simulink model "Senorless"  (R2023a)
settings: Solver=FixedStepDiscrete  StartTime=0.0  StopTime=2  FixedStep=1/FOC_FRQ  RelTol=1e-3
values from neighbouring files (symbols this model uses):
  ADC_REF = 3.6    [Senorless.sldd]
  ADC_SAMPLE_MAX = 32767.0    [Senorless.sldd]
  AMP_GAIN = 32.0    [Senorless.sldd]
  CURR_INPUT = 3276.0    [Senorless.sldd]
  CURR_KI = 380.0    [Senorless.sldd]
  CURR_KP = 0.04    [Senorless.sldd]
  CURR_LIMIT = 1.1    [Senorless.sldd]
  CURR_OVER = 34.0    [Senorless.sldd]
  CURR_POINT_GAIN = 7.0    [Senorless.sldd]
  CURR_STEP = 32760.0    [Senorless.sldd]
  CURR_UNDER = 0.03    [Senorless.sldd]
  CURR_WIDTH = 250.0    [Senorless.sldd]
  FOC_FRQ = 36000.0    [Senorless.sldd]
  GAMMA = 32767.0    [Senorless.sldd]
  HFI_ID = 2.125    [Senorless.sldd]
  IMAX = 34.0    [Senorless.sldd]
  LPF_FRQ = 300.0    [Senorless.sldd]
  MOTOR_DAMPER = 8.3E-7    [Senorless.sldd]
  MOTOR_FLUX = 0.0012713112    [Senorless.sldd]
  MOTOR_INERTIA = 1.02E-6    [Senorless.sldd]
  MOTOR_LS = 1.8E-5    [Senorless.sldd]
  MOTOR_PN = 7.0    [Senorless.sldd]
  MOTOR_RS = 0.065    [Senorless.sldd]
  NS_COMP_UD = 0.531    [Senorless.sldd]
  PLL_LIMIT = 0.95    [Senorless.sldd]
  PLL_WIDTH = 500.0    [Senorless.sldd]
  PWM_FRQ = 96000000.0    [Senorless.sldd]
  RS_HUNT = 0.002    [Senorless.sldd]
  SMOK_FRQ = 1200.0    [Senorless.sldd]
  SPD_LIMIT = 0.8    [Senorless.sldd]
  SPD_LPF_LEVEL = 15.0    [Senorless.sldd]
  SPD_MAX = 8100.0    [Senorless.sldd]
  SPD_MIN = -8100.0    [Senorless.sldd]
  SPD_REDUCE = 380.0    [Senorless.sldd]
  SPD_STEP = 3.0    [Senorless.sldd]
  SPD_WIDTH = 10.0    [Senorless.sldd]
  TS_POINT_GAIN = 10.0    [Senorless.sldd]
  UDC = 17.0    [Senorless.sldd]
  UDC_GAIN = 21.0    [Senorless.sldd]
  UDC_POINT_GAIN = 10.0    [Senorless.sldd]
undefined symbols (not defined in the file or in its folder): curr_q_ki, curr_q_kp, DiscIntNeverNeededParam, magnitude, PLL_LPF_LEVEL, Udc
libraries: simulink x20, slpidlib x5, mcbcontrolslib x4, mcbplantlib x1, autolibpmsminterior x1, autolibpmsmexterior x1, spspowerguiLib x1
(part 1 of 7)
settings Model: DataDictionary=Senorless.sldd  NumberOfSteps=10000  SnapshotBufferSize=5000  SnapshotInterval=5000  PacingRate=0.100000  Creator=lzm  LastModifiedBy=liangzhuoming
settings DataIOCC: SaveFormat=StructureWithTime  DSMLogging=off  ReturnWorkspaceOutputs=off
settings OptimizationCC: DefaultParameterBehavior=Inlined  GainParamInheritBuiltInType=on  UseFloatMulNetSlope=on  InheritOutputTypeSmallerThanSingle=on  DefaultUnderspecifiedDataType=single  UseSpecifiedMinMax=on  InlineInvariantSignals=on  StrengthReduction=on  PassReuseOutputArgsAs=Individual arguments  ZeroExternalMemoryAtStartup=off  ZeroInternalMemoryAtStartup=off  NoFixptDivByZeroProtection=on  EfficientFloat2IntCast=on  LifeSpan=1  OptimizeBlockOrder=speed  OptimizationPriority=Speed  MultiThreadedLoops=on  EfficientTunableParamExpr=on
settings DebuggingCC: SignalRangeChecking=warning  ParameterTunabilityLossMsg=error  UnconnectedInputMsg=warning  UnconnectedOutputMsg=warning  UnconnectedLineMsg=warning
settings HardwareCC: ProdBitPerPointer=32  ProdBitPerSizeT=32  ProdBitPerPtrDiffT=32  ProdLargestAtomicInteger=Long  ProdLargestAtomicFloat=Double  ProdWordSize=32  ProdLongLongMode=on  ProdHWDeviceType=ARM Compatible->ARM Cortex-M
settings ModelReferenceCC: EnableRefExpFcnMdlSchedulingChecks=on
settings SFSimCC: MATLABDynamicMemAlloc=off
settings RTWCC: Description=Embedded Coder  SystemTargetFile=ert.tlc  GenCodeOnly=on  TemplateMakefile=ert_default_tmf  GenerateReport=on  BuildConfiguration=Faster Runs  LaunchReport=on  GenerateCodeReplacementReport=on  DLArmComputeVersion=19.05
settings CodeAppCC: ForceParamTrailComments=on  IgnoreCustomStorageClasses=off  OperatorAnnotations=on  SimulinkDataObjDesc=on  SFDataObjDesc=on  CustomSymbolStrGlobalVar=rt$N$M  CustomSymbolStrType=$N$M  CustomSymbolStrFcn=$N$M$F  CustomSymbolStrMacro=$N$M  InsertBlockDesc=on
settings ERTTargetCC: TargetLangStandard=C99 (ISO)  GenerateSampleERTMain=on  IncludeMdlTerminateFcn=off  CombineSignalStateStructs=on  SupportNonFinite=off  SupportComplex=off  SupportNonInlinedSFcns=on  InlinedParameterPlacement=NonHierarchical  ERTCustomFileTemplate=example_file_process.tlc  ERTFilePackagingFormat=CompactWithDataFile

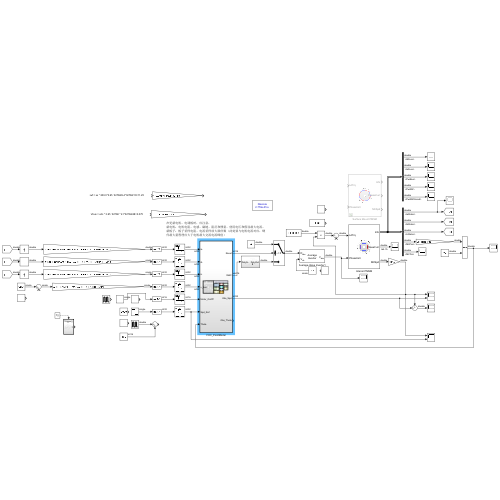
[thumbnail: Simulink's stored preview of the top-level diagram]
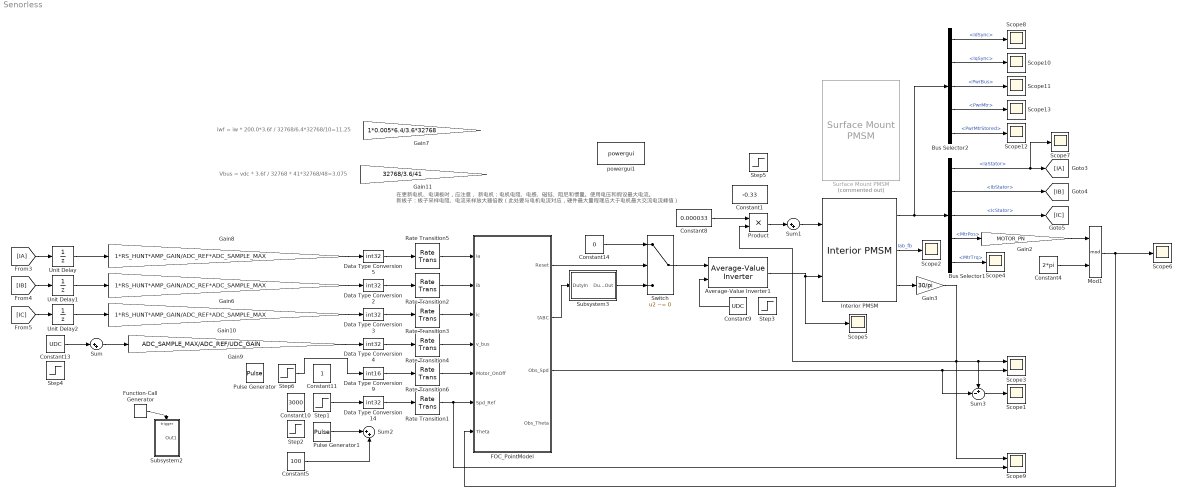
== system Senorless ==
  note: 在更新电机、电调板时，应注意，
      | 新电机：电机电阻、电感、磁链、阻尼和惯量。使用电压和假设最大电流。
      | 新板子：板子采样电阻、电流采样放大器倍数（此处要与电机电流对应，硬件最大量程理应大于电机最大交流电流峰值）
  note: iwf = iw * 200.0*3.6f / 32768/6.4*32768/10=11.25
  note: Vbus = vdc * 3.6f / 32768 * 41*32768/48=3.075
  Average-Value Inverter1 : mcbplantlib/Average-Value Inverter
  Bus Selector1 : BusSelector  OutputSignals=IaStator,IbStator,IcStator,MtrPos,MtrTrq
  Bus Selector2 : BusSelector  OutputSignals=IdSync,IqSync,PwrInfo.PwrTrnsfrd.PwrBus,PwrInfo.PwrTrnsfrd.PwrMtr,PwrInfo.PwrStored.PwrMtrStored
  Constant1 : Constant  Value=-0.33
  Constant10 : Constant  Value=3000  OutDataTypeStr=int16
  Constant11 : Constant
  Constant13 : Constant  Value=UDC  OutDataTypeStr=single
  Constant14 : Constant  Value=0
  Constant4 : Constant  Value=2*pi
  Constant5 : Constant  Value=100  OutDataTypeStr=int16
  Constant8 : Constant  Value=0.000033
  Constant9 : Constant  Value=UDC
  Data Type Conversion{2..5,14} (5 alike) : DataTypeConversion  OutDataTypeStr=int32  SaturateOnIntegerOverflow=off  RndMeth=Floor
  Data Type Conversion9 : DataTypeConversion  OutDataTypeStr=int16  SaturateOnIntegerOverflow=off  RndMeth=Floor
  FOC_PointModel : Subsystem  TreatAsAtomicUnit=on
      settings: RTWSystemCode=Nonreusable function
  Function-Call Generator : simulink/Ports & Subsystems/Function-Call Generator  sample_time=1/2500*100  numberOfIterations=1  DisallowWideOutput=off
  Gain10 : Gain  Gain=1*RS_HUNT*AMP_GAIN/ADC_REF*ADC_SAMPLE_MAX  OutDataTypeStr=single
  Gain11 : Gain  Gain=32768/3.6/41
  Gain2 : Gain  Gain=MOTOR_PN
  Gain3 : Gain  Gain=30/pi
  Gain6 : Gain  Gain=1*RS_HUNT*AMP_GAIN/ADC_REF*ADC_SAMPLE_MAX  OutDataTypeStr=single
  Gain7 : Gain  Gain=1*0.005*6.4/3.6*32768
  Gain8 : Gain  Gain=1*RS_HUNT*AMP_GAIN/ADC_REF*ADC_SAMPLE_MAX
  Gain9 : Gain  Gain=ADC_SAMPLE_MAX/ADC_REF/UDC_GAIN
  Interior PMSM : autolibpmsminterior/Interior PMSM  port_config=Torque  sim_type=Discrete  Ts=1/FOC_FRQ  FilePath=interiorpmsm_motordata.m  P=MOTOR_PN  Rs=MOTOR_RS  Ldq=[MOTOR_LS*0.7 MOTOR_LS/0.7]  KConstText=Permanent flux linkage constant (lambda_pm):  lambda_pm=MOTOR_FLUX  Ke=159.9771  mechanical=[MOTOR_INERTIA, MOTOR_DAMPER, 1e-6]  idq0=[0 0]  theta_init=1/MOTOR_PN*2*pi/360*0  omega_init=0  KConst=MOTOR_FLUX  lambda_pm_calc=MOTOR_FLUX  Kt=1.323  RefBlkName='autolibpmsminterior/Interior PMSM'  aMode=1
      settings: LibrarySourceBlock=autolibemachines/Interior PMSM
  Mod1 : Math  Operator=mod
  Product : Product
  Pulse Generator : DiscretePulseGenerator  PulseType=Time based  Period=1  PulseWidth=98
  Pulse Generator1 : DiscretePulseGenerator  PulseType=Time based  Amplitude=8100  Period=0.5  PulseWidth=90
  Rate Transition{1..6} (6 alike) : RateTransition
  Scope{1..2,4..8,10..13} (11 alike) : Scope
  Scope3 : Scope  NumInputPorts=2
  Scope9 : Scope  NumInputPorts=2
  Step1 : Step  Before=1000  After=-1000  OutDataTypeStr=single  SampleTime=0
  Step2 : Step  Time=1.5  After=8000  OutDataTypeStr=single  SampleTime=0
  Step3 : Step  Time=2.5  Before=48  After=47  OutDataTypeStr=single  SampleTime=0
  Step4 : Step  Time=2.5  Before=48  After=47  OutDataTypeStr=single  SampleTime=0
  Step5 : Step  Before=0.2  After=0  SampleTime=0
  Step6 : Step  Time=0.2  OutDataTypeStr=single  SampleTime=0
  Subsystem2 : Subsystem
  Subsystem3 : Subsystem
  Sum : Sum  Inputs=|++
  Sum1 : Sum  Inputs=|++
  Sum2 : Sum  Inputs=|++
  Sum3 : Sum  Inputs=+-|
  Surface Mount PMSM : autolibpmsmexterior/Surface Mount PMSM  Commented=on  port_config=Torque  sim_type=Discrete  Ts=1/FOC_FRQ  P=MOTOR_PN  Rs=MOTOR_RS  Ldq_=MOTOR_LS  KConstText=Permanent flux linkage constant (lambda_pm):  lambda_pm=MOTOR_FLUX  Ke=0.0059268  Kt=0.061  mechanical=[MOTOR_INERTIA, MOTOR_DAMPER, 0]  idq0=[0 0]  theta_init=4/5  omega_init=0  KConst=MOTOR_FLUX  lambda_pm_calc=MOTOR_FLUX  RefBlkName='autolibpmsmexterior/Surface Mount PMSM'  aMode=5  Ldq="[0.0017      0.0017]"
  Switch : Switch  Criteria=u2 ~= 0  SaturateOnIntegerOverflow=off  InputSameDT=off
  Unit Delay : UnitDelay  SampleTime=-1  HasFrameUpgradeWarning=on
  Unit Delay1 : UnitDelay  SampleTime=-1  HasFrameUpgradeWarning=on
  Unit Delay2 : UnitDelay  SampleTime=-1  HasFrameUpgradeWarning=on
  powergui1 : spspowerguiLib/powergui  Priority=1  SimulationMode=Discrete  SampleTime=1/FOC_FRQ  frequency=60  Iterations=50  frequencyindice=60  Pbase=100e6  ErrMax=1e-4  UnitsV=kV  UnitsW=MW  buscounter=0  FunctionMessages=off  echomessages=off  EnableUseOfTLC=off  CurrentSourceSwitches=off  DisableSnubberDevices=off  DisableRonSwitches=off  DisableVfSwitches=off  DisplayEquations=off  AutomaticDiscreteSolvers=off  SolverType=Tustin/Backward Euler (TBE)  Interpol=off  ExternalGateDelay=off  methode=off  Ts=100  x0status=blocks  SPID=on  SwTol=0  HookPort=off  NonlinearTolerance=1e-4  nMaxIteration=100  ContinueOnMaxIteration=off  RestoreLinks=warning  ResistiveCurrentMeasurement=off  Frange=[0:2:500]  Ylog=off  Xlog=on  ShowGrid=off  save=off  variable=ZData  structure=0  ZoomFFT=off  StartTime=0.0  cycles=1  DisplayStyle=1  fundamental=60  FreqAxis=off  MaxFrequency=1000  frequencyindicesteady=1  RmsSteady=1  display=off
  wires:
  Interior PMSM/3 -> Gain3/1
  Interior PMSM/2 -> Scope2/1  "Iab_fb"
  Interior PMSM/1 -> Bus Selector2/1, Bus Selector1/1
  Bus Selector1/1 -> Scope7/1, [IA]  "<IaStator>"
  Constant4/1 -> Mod1/2
  Gain2/1 -> Mod1/1
  Bus Selector1/4 -> Gain2/1  "<MtrPos>"
  Data Type Conversion5/1 -> Rate Transition5/1
  Data Type Conversion2/1 -> Rate Transition2/1
  Data Type Conversion3/1 -> Rate Transition3/1
  Data Type Conversion9/1 -> Rate Transition6/1
  [IC] -> Unit Delay2/1
  Gain8/1 -> Data Type Conversion5/1
  Gain6/1 -> Data Type Conversion2/1
  Gain10/1 -> Data Type Conversion3/1
  Gain9/1 -> Data Type Conversion4/1
  [IB] -> Unit Delay1/1
  [IA] -> Unit Delay/1
  FOC_PointModel/2(tABC) -> Subsystem3/1(DutyIn)
  Gain3/1 -> Scope9/1, Scope3/1, Sum3/1, Product/2
  Sum/1 -> Gain9/1
  Data Type Conversion4/1 -> Rate Transition4/1
  Mod1/1 -> FOC_PointModel/7(Theta), Scope6/1
  FOC_PointModel/3(Obs_Spd) -> Sum3/2, Scope3/2
  Data Type Conversion14/1 -> Rate Transition1/1
  Subsystem3/1(DutyOut) -> Switch/3
  Bus Selector1/5 -> Scope4/1  "<MtrTrq>"
  Average-Value Inverter1/1 -> Scope5/1, Interior PMSM/2
  FOC_PointModel/1(Reset) -> Switch/2
  Constant14/1 -> Switch/1
  Constant9/1 -> Average-Value Inverter1/2
  Constant13/1 -> Sum/1
  Rate Transition1/1 -> Scope9/2, FOC_PointModel/6(Spd_Ref)
  Function-Call Generator/1 -> Subsystem2/Trigger
  Rate Transition5/1 -> FOC_PointModel/1(ia)
  Rate Transition2/1 -> FOC_PointModel/2(ib)
  Rate Transition3/1 -> FOC_PointModel/3(ic)
  Rate Transition4/1 -> FOC_PointModel/4(v_bus)
  Rate Transition6/1 -> FOC_PointModel/5(Motor_OnOff)
  Constant5/1 -> Sum2/2
  Pulse Generator1/1 -> Sum2/1
  Constant8/1 -> Product/1
  Product/1 -> Sum1/1
  Bus Selector1/3 -> [IC]  "<IcStator>"
  Bus Selector1/2 -> [IB]  "<IbStator>"
  Switch/1 -> Average-Value Inverter1/1
  Sum3/1 -> Scope1/1
  Unit Delay/1 -> Gain8/1
  Unit Delay1/1 -> Gain6/1
  Unit Delay2/1 -> Gain10/1
  Bus Selector2/1 -> Scope8/1  "<IdSync>"
  Bus Selector2/2 -> Scope10/1  "<IqSync>"
  Bus Selector2/3 -> Scope11/1  "<PwrBus>"
  Bus Selector2/4 -> Scope13/1  "<PwrMtr>"
  Bus Selector2/5 -> Scope12/1  "<PwrMtrStored>"
  Step6/1 -> Data Type Conversion9/1
  Step1/1 -> Data Type Conversion14/1
  Sum1/1 -> Interior PMSM/1

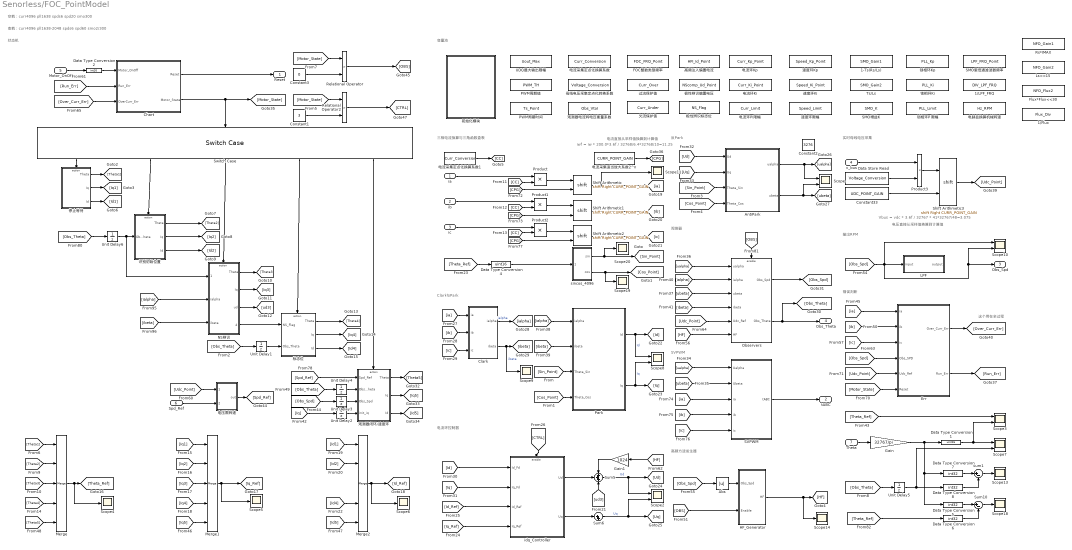
== system Senorless/FOC_PointModel ==
  note: 高频方波发生器
  note: 输出RPM
  note: 空载：curr4096 pll1638 spds6 spd20 smo300
  note: 这个用在全过程
  note: 错误判断
  note: 观测器
  note: SVPWM
  note: 反Park
  note: 实时母线电压采集
  note: 电流环控制器
  note: Clark与Park
  note: 三相电流换算与三角函数查表
  note: 变量池
  note: 状态机
  note: 电流直接从采样值换算到计算值
  note: Vbus = vdc * 3.6f / 32767 * 41*32767/48=3.075
  note: iwf = iw * 200.0*3.6f / 32768/6.4*32768/10=11.25
  note: 电压直接从采样值换算到计算值
  note: 变载：curr4096 pll1638-2048 spds6 spd60 smo2/300
  ia : Inport  OutDataTypeStr=int32
  ib : Inport  Port=2  OutDataTypeStr=int32
  ic : Inport  Port=3  OutDataTypeStr=int32
  v_bus : Inport  Port=4  OutDataTypeStr=int32
  Motor_OnOff : Inport  Port=5
  Spd_Ref : Inport  Port=6
  Theta : Inport  Port=7
  1-Ts(Rs/Ls) : DataStoreMemory  DataStoreName=SMO_Gain1  WriteAfterWriteMsg=warning  ShowAdditionalParam=off
  1/Flux : DataStoreMemory  DataStoreName=Flux_Div  WriteAfterWriteMsg=warning  ShowAdditionalParam=off
  1/LPF_FRQ : DataStoreMemory  DataStoreName=DIV_LPF_FRQ  WriteAfterWriteMsg=warning  ShowAdditionalParam=off
  Abs : Abs  SaturateOnIntegerOverflow=off
  AntiPark : Subsystem
  Chart : Stateflow chart  TreatAsAtomicUnit=on
  Clark : Subsystem
  Constant1 : Constant  Value=3  OutDataTypeStr=uint8
  Constant2 : Constant  Value=3276  OutDataTypeStr=int16
  Constant3 : Constant  Value=0  OutDataTypeStr=uint8
  Constant33 : Constant  Value=UDC_POINT_GAIN
  Data Store Read : DataStoreRead  DataStoreName=Voltage_Conversion  IndexOptions=Index vector (dialog)  Indices=1  OutputSizes=1
  Data Type Conversion1 : DataTypeConversion  OutDataTypeStr=uint16  SaturateOnIntegerOverflow=off  RndMeth=Floor
  Data Type Conversion2 : DataTypeConversion  OutDataTypeStr=int16  SaturateOnIntegerOverflow=off
  Data Type Conversion4 : DataTypeConversion  OutDataTypeStr=uint16  SaturateOnIntegerOverflow=off
  Data Type Conversion{5..8} (4 alike) : DataTypeConversion  OutDataTypeStr=int32  SaturateOnIntegerOverflow=off
  Err : Subsystem
  FOC整数类型频率 : DataStoreMemory  DataStoreName=FOC_FRQ_Point  WriteAfterWriteMsg=warning  ShowAdditionalParam=off
  Flux*Flux<<30 : DataStoreMemory  DataStoreName=NFO_Flux2  WriteAfterWriteMsg=warning  ShowAdditionalParam=off
  Gain : Gain  Gain=32767/pi
  Gain1 : Gain  Gain=1024  ParamDataTypeStr=int16  OutDataTypeStr=int16  RndMeth=Zero
  HF_Generator : Subsystem
  LPF : Subsystem  TreatAsAtomicUnit=on
  Ls<<15 : DataStoreMemory  DataStoreName=NFO_Gain2  WriteAfterWriteMsg=warning  ShowAdditionalParam=off
  Merge : Merge  Inputs=5
  Merge1 : Merge  Inputs=5
  Merge2 : Merge  Inputs=5
  NS辨识 : Subsystem  TreatAsAtomicUnit=on
  Observers : Subsystem
  PWM周期值 : DataStoreMemory  DataStoreName=PWM_TH  WriteAfterWriteMsg=warning  ShowAdditionalParam=off
  PWM周期时间 : DataStoreMemory  DataStoreName=Ts_Point  WriteAfterWriteMsg=warning  ShowAdditionalParam=off
  Park : Subsystem
  Product{,1..3} (4 alike) : Product  OutDataTypeStr=int32  RndMeth=Zero
  Relational Operator : RelationalOperator  Operator=>  OutDataTypeStr=boolean  RndMeth=Zero  InputSameDT=off
  Relational Operator2 : RelationalOperator  Operator=>  OutDataTypeStr=boolean  RndMeth=Zero  InputSameDT=off
  Rs*IMAX : DataStoreMemory  DataStoreName=NFO_Gain1  WriteAfterWriteMsg=warning  ShowAdditionalParam=off
  SMO增益K : DataStoreMemory  DataStoreName=SMO_K  WriteAfterWriteMsg=warning  ShowAdditionalParam=off
  SMO里低通滤波器频率 : DataStoreMemory  DataStoreName=LPF_FRQ_Point  WriteAfterWriteMsg=warning  ShowAdditionalParam=off
  SVPWM : Subsystem  ScheduleAs=Aperiodic partition  PartitionName=TEMP_PRECOMP_PARTITION_NAME_MessageTriggeredSubsystem
  Scope{,2..3,7..8,10} (6 alike) : Scope  NumInputPorts=2
  Scope{4..6,9,11,13..14,18..20} (10 alike) : Scope
  Shift Arithmetic{,1..3} (4 alike) : ArithShift  BitShiftNumberSource=Input port  BitShiftNumber=CURR_POINT_GAIN  BitShiftDirection=Right
      settings: InputPortMap=u0,p1
  Sum1 : Sum  Inputs=|+-  OutDataTypeStr=int32
  Sum10 : Sum  Inputs=|+-  OutDataTypeStr=int32
  Sum5 : Sum  Inputs=+++
  Sum6 : Sum  Inputs=|++
  Switch Case : SwitchCase  CaseConditions={0,1,2,3,4}  ShowDefaultCase=off
  Ts/Ls : DataStoreMemory  DataStoreName=SMO_Gain2  WriteAfterWriteMsg=warning  ShowAdditionalParam=off
  UDQ最大输出限幅 : DataStoreMemory  DataStoreName=Uout_Max  WriteAfterWriteMsg=warning  ShowAdditionalParam=off
  Unit Delay{1..6} (6 alike) : UnitDelay  SampleTime=-1  HasFrameUpgradeWarning=on
  idq_Controller : Subsystem
  sincos_4096 : Subsystem
  停止等待 : Subsystem  TreatAsAtomicUnit=on
  初始化模块 : Subsystem  TreatAsAtomicUnit=on
  极性辨识偏置电压 : DataStoreMemory  DataStoreName=NScomp_Ud_Point  WriteAfterWriteMsg=warning  ShowAdditionalParam=off
  极性辨识标志位 : DataStoreMemory  DataStoreName=NS_Flag  WriteAfterWriteMsg=warning  ShowAdditionalParam=off
  标志位 : Subsystem  TreatAsAtomicUnit=on
  欠流保护值 : DataStoreMemory  DataStoreName=Curr_Under  WriteAfterWriteMsg=warning  ShowAdditionalParam=off
  母线电压采集定点化转换系数 : DataStoreMemory  DataStoreName=Voltage_Conversion  WriteAfterWriteMsg=warning  ShowAdditionalParam=off
  电压限转速 : Subsystem
  电流环Ki : DataStoreMemory  DataStoreName=Curr_Ki_Point  WriteAfterWriteMsg=warning  ShowAdditionalParam=off
  电流环Kp : DataStoreMemory  DataStoreName=Curr_Kp_Point  WriteAfterWriteMsg=warning  ShowAdditionalParam=off
  电流环PI限幅 : DataStoreMemory  DataStoreName=Curr_Limit  WriteAfterWriteMsg=warning  ShowAdditionalParam=off
  电流采集定点化换算系数 : DataStoreMemory  DataStoreName=Curr_Conversion  WriteAfterWriteMsg=warning  ShowAdditionalParam=off
  电流采集定点化换算系数1 : DataStoreRead  DataStoreName=Curr_Conversion  IndexOptions=Index vector (dialog)  Indices=1  OutputSizes=1
  电流采集适当放大系数2^n : Constant  Value=CURR_POINT_GAIN
  电赫兹换算机械转速 : DataStoreMemory  DataStoreName=Hz_RPM  WriteAfterWriteMsg=warning  ShowAdditionalParam=off
  观测器电流转电压衡量系数 : DataStoreMemory  DataStoreName=Obs_VtoI  WriteAfterWriteMsg=warning  ShowAdditionalParam=off
  观测器闭环/速度环 : Subsystem  TreatAsAtomicUnit=on
  识别初始位置 : Subsystem  TreatAsAtomicUnit=on
  过流保护值 : DataStoreMemory  DataStoreName=Curr_Over  WriteAfterWriteMsg=warning  ShowAdditionalParam=off
  速度环Ki : DataStoreMemory  DataStoreName=Speed_Ki_Point  WriteAfterWriteMsg=warning  ShowAdditionalParam=off
  速度环Kp : DataStoreMemory  DataStoreName=Speed_Kp_Point  WriteAfterWriteMsg=warning  ShowAdditionalParam=off
  速度环限幅 : DataStoreMemory  DataStoreName=Speed_Limit  WriteAfterWriteMsg=warning  ShowAdditionalParam=off
  锁相环Ki : DataStoreMemory  DataStoreName=PLL_Ki  WriteAfterWriteMsg=warning  ShowAdditionalParam=off
  锁相环Kp : DataStoreMemory  DataStoreName=PLL_Kp  WriteAfterWriteMsg=warning  ShowAdditionalParam=off
  锁相环PI限幅 : DataStoreMemory  DataStoreName=PLL_Limit  WriteAfterWriteMsg=warning  ShowAdditionalParam=off
  高频注入偏置电流 : DataStoreMemory  DataStoreName=HFI_Id_Point  WriteAfterWriteMsg=warning  ShowAdditionalParam=off
  Reset : Outport
  tABC : Outport  Port=2
  Obs_Spd : Outport  Port=3
  Obs_Theta : Outport  Port=4
  wires:
  Motor_OnOff/1 -> Data Type Conversion2/1
  Switch Case/1 -> 停止等待/Action
  Switch Case/3 -> NS辨识/Action
  Switch Case/2 -> 识别初始位置/Action
  Switch Case/4 -> 标志位/Action
  [Sin_Point] -> AntiPark/3(Theta_Sin)
  [Cos_Point] -> AntiPark/4(Theta_Cos)
  v_bus/1 -> Product3/1
  Product1/1 -> Shift Arithmetic1/1
  Product2/1 -> Shift Arithmetic2/1
  电流采集定点化换算系数1/1 -> [CC]
  [CC] -> Product/2
  [CC] -> Product1/2
  Data Store Read/1 -> Product3/2
  Unit Delay1/1 -> 标志位/2(Obs_Theta)
  停止等待/1(Theta) -> [Theta1]
  停止等待/2(Iq) -> [Iq1]
  停止等待/3(Id) -> [Id1]
  识别初始位置/1(Theta) -> [Theta2]
  识别初始位置/2(Iq) -> [Iq2]
  识别初始位置/3(Id) -> [Id2]
  标志位/2(Iq) -> [Iq4]
  标志位/3(Id) -> [Id4]
  [Theta1] -> Merge/1
  [Theta3] -> Merge/3
  [Theta4] -> Merge/4
  [Iq1] -> Merge1/1
  [Iq2] -> Merge1/2
  [Iq3] -> Merge1/3
  [Iq4] -> Merge1/4
  Merge1/1 -> [Iq_Ref], Scope5/1
  [Id1] -> Merge2/1
  [Id2] -> Merge2/2
  [Id4] -> Merge2/4
  [Iq_Ref] -> idq_Controller/4(Iq_Ref)
  Shift Arithmetic/1 -> [ia], Scope11/1
  Shift Arithmetic1/1 -> [ib]
  Shift Arithmetic2/1 -> [ic]
  [ia] -> Clark/1(ia)
  [ib] -> Clark/2(ib)
  [ic] -> Clark/3(ic)
  [Iq] -> idq_Controller/2(Iq_Fd)
  [Id] -> idq_Controller/1(Id_Fd)
  [ualpha] -> SVPWM/1(Ualpha)
  [ubeta] -> SVPWM/2(Ubeta)
  Clark/1(ialpha) -> [ialpha]  "ialpha"
  Clark/2(ibeta) -> Scope9/1, [ibeta]  "ibeta"
  [ualpha] -> Observers/1(ualpha)
  [ibeta] -> Observers/4(ibeta)
  [ubeta] -> Observers/3(ubeta)
  [ialpha] -> Observers/2(ialpha)
  标志位/1(Theta) -> [Theta4]
  Observers/2(Obs_Theta) -> Obs_Theta/1, [Obs_Theta]
  Switch Case/5 -> 观测器闭环/速度环/Action
  观测器闭环/速度环/2(Iq) -> [Iq5]
  观测器闭环/速度环/3(Id) -> [Id5]
  [Iq5] -> Merge1/5
  [Id5] -> Merge2/5
  Theta/1 -> Gain/1
  [Theta5] -> Merge/5
  Gain/1 -> Data Type Conversion5/1, Data Type Conversion7/1, Data Type Conversion1/1
  [Theta_Ref] -> Data Type Conversion4/1
  Chart/2(Motor_State) -> Switch Case/1, [Motor_State]
  Merge/1 -> Scope4/1, [Theta_Ref]
  Sum1/1 -> Scope13/1
  Data Type Conversion7/1 -> Sum1/1
  Data Type Conversion8/1 -> Sum1/2
  [Obs_Theta] -> Unit Delay5/1
  [CC] -> Product2/2
  Product3/1 -> Shift Arithmetic3/1
  Constant33/1 -> Shift Arithmetic3/2
  [Theta_Ref] -> Scope3/1
  [Obs_Spd] -> Unit Delay3/1
  [Run_Err] -> Chart/2(Run_Err)
  SVPWM/1(tABC) -> tABC/1
  Chart/1(Reset) -> Reset/1
  [Obs_Theta] -> Unit Delay4/1
  Unit Delay3/1 -> 观测器闭环/速度环/3(Obs_Spd)
  Shift Arithmetic3/1 -> [Udc_Point]
  [Udc_Point] -> 电压限转速/1(Udc_Ref)
  [Over_Curr_Err] -> Chart/3(OverCurr_Err)
  ia/1 -> Product/1
  ic/1 -> Product2/1
  Data Type Conversion2/1 -> Chart/1(Motor_OnOff)
  Sum5/1 -> [Ud], Scope2/1  "Ud"
  [ia] -> Err/1(ia)
  [ib] -> Err/2(ib)
  [ic] -> Err/3(ic)
  [Obs_Spd] -> Err/4(Obs_SPD)
  Err/1(Over_Curr_Err) -> [Over_Curr_Err]
  Err/2(Run_Err) -> [Run_Err]
  [Motor_State] -> Err/6(Reset)
  [Udc_Point] -> Observers/5(Udc_Ref)
  [Udc_Point] -> Err/5(Udc_Ref)
  AntiPark/1(ualpha) -> Scope/1, [ualpha]
  AntiPark/2(ubeta) -> Scope/2, [ubeta]
  [ia] -> SVPWM/3(ia)
  [ib] -> SVPWM/4(ib)
  [ic] -> SVPWM/5(ic)
  [CPG] -> Shift Arithmetic/2
  [CPG] -> Shift Arithmetic1/2
  [CPG] -> Shift Arithmetic2/2
  Product/1 -> Shift Arithmetic/1
  电流采集适当放大系数2^n/1 -> [CPG]
  Relational Operator/1 -> [OBS]
  [Motor_State] -> Relational Operator/1
  Constant3/1 -> Relational Operator/2
  Park/1(Id) -> Scope8/1, [Id]  "Id"
  Park/2(Iq) -> Scope8/2, [Iq]  "Iq"
  [ialpha] -> Park/1(ialpha)
  [ibeta] -> Park/2(ibeta)
  [Sin_Point] -> Park/3(Theta_Sin)
  [Cos_Point] -> Park/4(Theta_Cos)
  Unit Delay5/1 -> Data Type Conversion8/1, Scope7/2
  ib/1 -> Product1/1
  Data Type Conversion6/1 -> Sum10/2
  Data Type Conversion5/1 -> Sum10/1
  [Theta_Ref] -> Data Type Conversion6/1
  Sum10/1 -> Scope18/1
  Data Type Conversion4/1 -> sincos_4096/1(theta)
  sincos_4096/2(cos) -> Scope19/1, [Cos_Point]
  sincos_4096/1(sin) -> Scope20/1, [Sin_Point]
  [Obs_Spd] -> LPF/1(input), Scope10/2, Obs_Spd/1, Scope10/1
  [Ud] -> AntiPark/1(Ud)
  [HF] -> Gain1/1
  idq_Controller/2(Uq) -> Sum6/1
  Spd_Ref/1 -> 电压限转速/2(SPD_Ref)
  [HF] -> Observers/6(HF)
  Observers/1(Obs_Spd) -> [Obs_Spd]
  电压限转速/1(out) -> [Spd_Ref]
  [Obs_Spd] -> Abs/1
  NS辨识/1(Theta) -> [Theta3]
  NS辨识/2(Iq) -> [Iq3]
  观测器闭环/速度环/1(Theta) -> [Theta5]
  Unit Delay4/1 -> 观测器闭环/速度环/2(Obs_Theta)
  [Theta2] -> Merge/2
  [Uq] -> AntiPark/2(Uq)
  Sum6/1 -> [Uq], Scope2/2  "Uq"
  HF_Generator/1(HF) -> Scope14/1, [HF]
  idq_Controller/1(Ud) -> Sum5/2
  Unit Delay6/1 -> NS辨识/1(Obs_Theta), 识别初始位置/1(Obs_Theta)
  Data Type Conversion1/1 -> Scope3/2, Scope7/1
  [Id_Ref] -> idq_Controller/3(Id_Ref)
  NS辨识/3(ud) -> [ud3]
  Gain1/1 -> Sum5/1
  Merge2/1 -> [Id_Ref], Scope6/1
  [Obs_Theta] -> Unit Delay6/1
  [ialpha] -> NS辨识/2(ialpha)
  [ibeta] -> NS辨识/3(ibeta)
  NS辨识/4(NS_Flag) -> 标志位/1(NS_Flag)
  [Obs_Theta] -> Unit Delay1/1
  [OBS] -> Observers/Enable
  Constant1/1 -> Relational Operator2/2
  [Motor_State] -> Relational Operator2/1
  Relational Operator2/1 -> [CTRL]
  [CTRL] -> idq_Controller/Enable
  [ud3] -> Sum5/3
  Abs/1 -> HF_Generator/1(Obs_Spd)
  [Iq] -> Unit Delay2/1
  Unit Delay2/1 -> 观测器闭环/速度环/4(init_iq)
  [Spd_Ref] -> 观测器闭环/速度环/1(Spd_Ref)
  [OBS] -> HF_Generator/2(Enable)

== system Senorless/Subsystem2 ==
  Trigger : TriggerPort  TriggerType=function-call  VariantControl=(inherit)  PortDimensions=1
  Constant1 : Constant  Value=0.25  OutDataTypeStr=single
  Constant16 : Constant  Value=SPD_MAX
  Product2 : Product
  Random Number1 : RandomNumber  Mean=0.1  Variance=0.01  Seed=15
  Saturation1 : Saturate  UpperLimit=1  LowerLimit=0
  Scope : Scope  NumInputPorts=2
  Sum : Sum  Inputs=|++
  Out1 : Outport
  wires:
  Saturation1/1 -> Product2/1
  Constant16/1 -> Product2/2
  Product2/1 -> Out1/1
  Sum/1 -> Scope/2, Saturation1/1
  Random Number1/1 -> Scope/1, Sum/1
  Constant1/1 -> Sum/2

== system Senorless/Subsystem3 ==
  DutyIn : Inport
  Constant : Constant  Value=0.5  SampleTime=-1
  Constant1 : Constant  SampleTime=-1
  Constant7 : Constant  Value=PWM_FRQ
  Constant8 : Constant  Value=FOC_FRQ*2
  Display : Display
  Divide : Product  Inputs=*/
  Divide1 : Product  Inputs=*/
  Divide2 : Product  Inputs=*/
  DutyIn1 : InportShadow
  Gain1 : Gain  Gain=-1
  Product : Product
  Scope : Scope  NumInputPorts=2
  Sum : Sum  Inputs=|+-
  Sum1 : Sum  Inputs=|++
  DutyOut : Outport
  wires:
  Divide/1 -> Product/1, Display/1
  Constant1/1 -> Divide/1
  Divide2/1 -> Divide1/2, Divide/2
  Constant7/1 -> Divide2/1
  Constant8/1 -> Divide2/2
  Product/1 -> Sum/1
  Sum1/1 -> DutyOut/1, Scope/2
  Gain1/1 -> Sum1/1
  DutyIn/1 -> Product/2
  Constant/1 -> Sum/2, Sum1/2
  Sum/1 -> Gain1/1
  Divide1/1 -> Scope/1
  DutyIn1/1 -> Divide1/1

== system Senorless/FOC_PointModel/AntiPark ==
  note: Valpha = ud*cos(theta) - uq*sin(theta);
      | Vbeta = ud*sin(theta) + uq*cos(theta);
  Ud : Inport
  Uq : Inport  Port=2
  Theta_Sin : Inport  Port=3
  Theta_Cos : Inport  Port=4
  Add : Sum  Inputs=+-  OutDataTypeStr=int32
  Add1 : Sum  OutDataTypeStr=int32
  Product{,1..3} (4 alike) : Product  OutDataTypeStr=int32  RndMeth=Zero
  Shift Arithmetic : ArithShift  BitShiftNumber=15  DiagnosticForOORShift=Error
  Shift Arithmetic1 : ArithShift  BitShiftNumber=15  DiagnosticForOORShift=Error
  Theta_Cos1 : InportShadow  Port=4
  Theta_Sin1 : InportShadow  Port=3
  Ud1 : InportShadow
  Uq1 : InportShadow  Port=2
  ualpha : Outport
  ubeta : Outport  Port=2
  wires:
  Theta_Cos/1 -> Product/2
  Ud/1 -> Product/1
  Add/1 -> Shift Arithmetic/1
  Shift Arithmetic/1 -> ualpha/1
  Shift Arithmetic1/1 -> ubeta/1
  Product1/1 -> Add/2
  Product/1 -> Add/1
  Uq/1 -> Product1/1
  Theta_Sin/1 -> Product1/2
  Add1/1 -> Shift Arithmetic1/1
  Product2/1 -> Add1/1
  Product3/1 -> Add1/2
  Ud1/1 -> Product2/1
  Theta_Sin1/1 -> Product2/2
  Theta_Cos1/1 -> Product3/2
  Uq1/1 -> Product3/1

== system Senorless/FOC_PointModel/Clark ==
  note: ialpha = ia;
      | ibeta = (ib-ic)/sqrt(3);
  ia : Inport
  ib : Inport  Port=2
  ic : Inport  Port=3
  Add2 : Sum  Inputs=+-  OutDataTypeStr=int32  RndMeth=Zero
  Gain2 : Gain  Gain=32767/sqrt(3)  ParamDataTypeStr=int16  OutDataTypeStr=int32  RndMeth=Zero
  Shift Arithmetic : ArithShift  BitShiftNumber=15  DiagnosticForOORShift=Error
  ialpha : Outport
  ibeta : Outport  Port=2
  wires:
  Gain2/1 -> Shift Arithmetic/1
  Add2/1 -> Gain2/1
  ic/1 -> Add2/2
  ib/1 -> Add2/1
  Shift Arithmetic/1 -> ibeta/1
  ia/1 -> ialpha/1

== system Senorless/FOC_PointModel/Err ==
  ia : Inport
  ib : Inport  Port=2
  ic : Inport  Port=3
  Obs_SPD : Inport  Port=4
  Udc_Ref : Inport  Port=5
  Reset : Inport  Port=6
  Abs1 : Abs  RndMeth=Zero  SaturateOnIntegerOverflow=off
  Abs2 : Abs  RndMeth=Zero  SaturateOnIntegerOverflow=off
  Abs3 : Abs  RndMeth=Zero  SaturateOnIntegerOverflow=off
  Data Store Read3 : DataStoreRead  DataStoreName=Curr_Over  IndexOptions=Index vector (dialog)  Indices=1  OutputSizes=1
  Max : MinMax  Function=max  Inputs=3  RndMeth=Zero
  PLL_LPF1 : Subsystem  TreatAsAtomicUnit=on
  Relational Operator : RelationalOperator  Operator=<  OutDataTypeStr=boolean  RndMeth=Zero  InputSameDT=off
  Relational Operator1 : RelationalOperator  Operator===  OutDataTypeStr=boolean  RndMeth=Zero  InputSameDT=off
  Scope : Scope
  Unit Delay : UnitDelay  SampleTime=-1  HasFrameUpgradeWarning=on
  闭环是4 : Constant  Value=4  OutDataTypeStr=uint8
  闭环错误判断 : Subsystem
  Over_Curr_Err : Outport
  Run_Err : Outport  Port=2
  wires:
  Abs2/1 -> Max/2
  Abs3/1 -> Max/3
  Data Store Read3/1 -> Relational Operator/1
  PLL_LPF1/1(output) -> Scope/1, 闭环错误判断/2(Curr_Max), Relational Operator/2
  Abs1/1 -> Max/1
  Max/1 -> PLL_LPF1/1(input)
  Relational Operator/1 -> 闭环错误判断/1(Curr_Err), Over_Curr_Err/1
  ic/1 -> Abs3/1
  ia/1 -> Abs1/1
  ib/1 -> Abs2/1
  Obs_SPD/1 -> 闭环错误判断/3(Obs_SPD)
  Udc_Ref/1 -> 闭环错误判断/4(Udc_Ref)
  闭环错误判断/1(Run_Err) -> Run_Err/1
  闭环是4/1 -> Relational Operator1/2
  Relational Operator1/1 -> 闭环错误判断/Enable
  Reset/1 -> Unit Delay/1
  Unit Delay/1 -> Relational Operator1/1

== system Senorless/FOC_PointModel/HF_Generator ==
  note: 1000-1500是缓冲段，虽然OBS没用到HFI，但他可以先开始工作
  note: 目前，低速开启方波，转速升高到1500以上关闭方波。从高转速下降小于1000转速会开启方波。
  Obs_Spd : Inport
  Enable : Inport  Port=2
  Chart : Stateflow chart  TreatAsAtomicUnit=on
  Constant5 : Constant  OutDataTypeStr=int16
  Constant6 : Constant  Value=0  OutDataTypeStr=int16
  Logical Operator : Logic  AllPortsSameDT=off  OutDataTypeStr=boolean
  Pulse Generator1 : DiscretePulseGenerator  Amplitude=int16(2)  SampleTime=-1
  Sum2 : Sum  Inputs=+-
  Switch : Switch  Criteria=u2 > Threshold  SaturateOnIntegerOverflow=off  InputSameDT=off
  Unit Delay : UnitDelay  SampleTime=-1  HasFrameUpgradeWarning=on
  HF : Outport
  wires:
  Constant6/1 -> Switch/3
  Sum2/1 -> Switch/1
  Switch/1 -> HF/1
  Obs_Spd/1 -> Unit Delay/1
  Pulse Generator1/1 -> Sum2/1
  Constant5/1 -> Sum2/2
  Logical Operator/1 -> Switch/2
  Unit Delay/1 -> Chart/1(Obs_SPD)
  Enable/1 -> Logical Operator/2
  Chart/1(output) -> Logical Operator/1

== system Senorless/FOC_PointModel/LPF ==
  note: a =(ω c​ T s​ )/(1+ω c​ T s​ )
  note: y(n)=ax(n)+(1−a)y(n−1)
  input : Inport
  Constant1 : Constant  Value=0  OutDataTypeStr=int16
  Constant5 : Constant  OutDataTypeStr=int16
  Product10 : Product  OutDataTypeStr=int32
  Product11 : Product  OutDataTypeStr=int32  RndMeth=Zero
  Saturation : Saturate  UpperLimit=15  LowerLimit=0  RndMeth=Zero
  Shift Arithmetic1 : ArithShift  BitShiftNumber=-4
  Shift Arithmetic9 : ArithShift  BitShiftNumber=4
  Sum10 : Sum  Inputs=-+
  Sum11 : Sum  OutDataTypeStr=int32  RndMeth=Zero
  Unit Delay9 : UnitDelay  SampleTime=-1  HasFrameUpgradeWarning=on
  output : Outport
  wires:
  Constant1/1 -> Saturation/1
  Constant5/1 -> Shift Arithmetic1/1
  Sum11/1 -> Shift Arithmetic9/1
  Shift Arithmetic9/1 -> output/1, Unit Delay9/1
  Shift Arithmetic1/1 -> Sum10/2
  Sum10/1 -> Product10/1
  Product11/1 -> Sum11/1
  Product10/1 -> Sum11/2
  Unit Delay9/1 -> Product11/1
  input/1 -> Product10/2
  Saturation/1 -> Sum10/1, Product11/2

== system Senorless/FOC_PointModel/NS辨识 ==
  Obs_Theta : Inport
  ialpha : Inport  Port=2
  ibeta : Inport  Port=3
  Action Port : ActionPort  InitializeStates=reset  ActionPortLabel=case [ 2 ]:
  Abs : Abs  SaturateOnIntegerOverflow=off
  Add2 : Sum
  Constant1 : Constant  Value=0  OutDataTypeStr=int16
  Data Store Read : DataStoreRead  DataStoreName=NScomp_Ud_Point  IndexOptions=Index vector (dialog)  Indices=1  OutputSizes=1
  Delay2 : Delay  DelayLength=1
  Obs_Theta1 : InportShadow
  Product4 : Product  OutDataTypeStr=int32  RndMeth=Zero
  Product5 : Product  OutDataTypeStr=int32  RndMeth=Zero
  Shift Arithmetic4 : ArithShift  BitShiftNumber=15  DiagnosticForOORShift=Error
  Sign : Signum
  Sum : Sum  Inputs=+-
  Sum2 : Sum  Inputs=|+-
  Unary Minus : UnaryMinus
  max : Subsystem
  min : Subsystem
  sincos_4096 : Subsystem
  加速积分角度 : Subsystem  Commented=on
  正负偏置 : Stateflow chart  TreatAsAtomicUnit=on
  Theta : Outport
  Iq : Outport  Port=2
  ud : Outport  Port=3
  NS_Flag : Outport  Port=4
  wires:
  Constant1/1 -> Iq/1
  Obs_Theta/1 -> Theta/1
  Obs_Theta1/1 -> sincos_4096/1(theta)
  Product5/1 -> Add2/2
  Product4/1 -> Add2/1
  Delay2/1 -> Sum2/2
  Add2/1 -> Shift Arithmetic4/1
  Sum2/1 -> Abs/1
  Abs/1 -> min/1(input), max/1(input)
  Sign/1 -> Unary Minus/1, max/Enable
  Unary Minus/1 -> min/Enable
  max/1(output) -> Sum/1
  min/1(output) -> Sum/2
  Sum/1 -> NS_Flag/1
  正负偏置/1(output) -> Sign/1, ud/1
  Data Store Read/1 -> 正负偏置/1(comp)
  ibeta/1 -> Product5/2
  ialpha/1 -> Product4/1
  sincos_4096/1(cos) -> Product4/2
  sincos_4096/2(sin) -> Product5/1
  Shift Arithmetic4/1 -> Delay2/1, Sum2/1

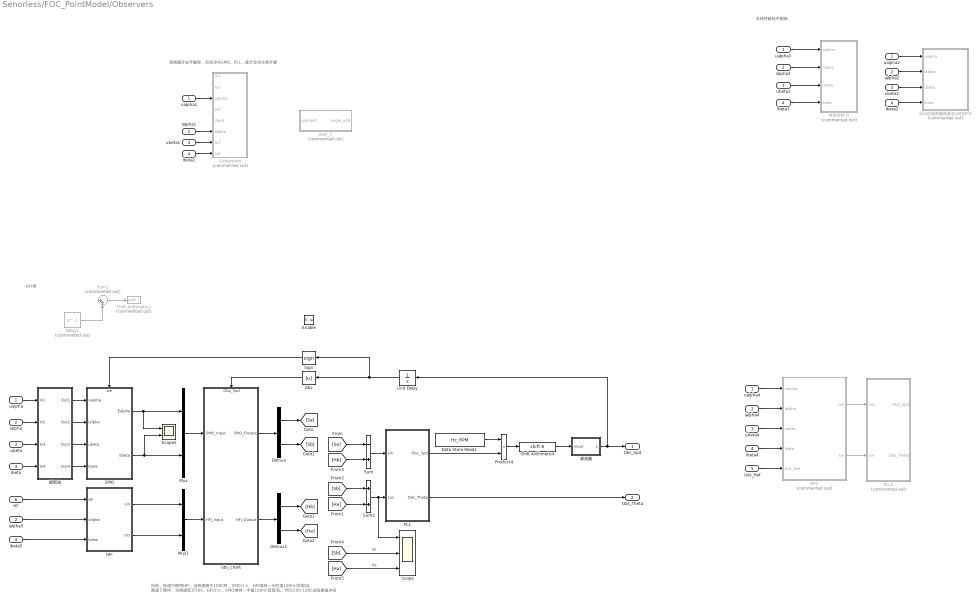
== system Senorless/FOC_PointModel/Observers ==
  note: 非线性磁链手脚架
  note: 观测器开发手脚架，包含浮点SMO、PLL，逐步定点化等步骤
  note: HFI用
  note: 目前，低速只使用HFI，当转速高于1000时，SMO介入，HFI维持一半的值100ms后取消。
      | 高速下降时，当转速低于500，HFI介入，SMO维持一半值100ms后取消。
      |
      | 所以500-1000这段是缓冲段
  ualpha : Inport
  ialpha : Inport  Port=2
  ubeta : Inport  Port=3
  ibeta : Inport  Port=4
  Udc_Ref : Inport  Port=5
  HF : Inport  Port=6
  Enable : EnablePort  StatesWhenEnabling=reset
  Abs : Abs  SaturateOnIntegerOverflow=off
  Data Store Read1 : DataStoreRead  DataStoreName=Hz_RPM  IndexOptions=Index vector (dialog)  Indices=1  OutputSizes=1
  Delay1 : Delay  Commented=on  DelayLength=1
  Demux : Demux  Outputs=2
  Demux1 : Demux  Outputs=2
  HFI : Subsystem  TreatAsAtomicUnit=on
  Mux : Mux  Inputs=2
  Mux1 : Mux  Inputs=2
  NFO : Subsystem  Commented=on
  PLL : Subsystem  TreatAsAtomicUnit=on
  PLL2 : Subsystem  Commented=on  TreatAsAtomicUnit=on
  Product4 : Product  OutDataTypeStr=int32  RndMeth=Zero
  SMO : Subsystem  TreatAsAtomicUnit=on
      settings: PortSchema="{\"entries\":[{\"content\":{\"sides\":[{\"content\":{\"connectorIds\":[\"In1\",\"In2\",\"In3\",\"In4\"]},\"type\":\"ConnectorPlacement.EquallySpacedRectSide\",\"uuid\":\"5d41c110-b961-4805-9997-4ea01628d80e\"},{\"content\":{\"connectorIds\":[\"Out1\",\"Out2\"],\"side\":\"RIGHT\"},\"type\":\"ConnectorPlacement.EquallySpacedRectSide\",\"uuid\":\"4de46d9b-8730-4f38-ad6a-6c44e7153813\"},{\"content\":{\"connectorIds\":[\"In5\"],\"side\":\"TOP\"},\"type\":\"ConnectorPlacement.EquallySpacedRectSide\",\"uuid\":\"5860a50a-79c2-4856-8676-a27b80772c77\"}]},\"type\":\"ConnectorPlacement.EquallySpacedConnector\",\"uuid\":\"397b29b2-225c-47ad-b447-1982dcf95bf6\"}],\"packageUris\":[\"http://schema.mathworks.com/mf0/Connector/R2020b\"],\"version\":\"1.0\"}"
  Scope : Scope  NumInputPorts=3
  Scope2 : Scope  NumInputPorts=2
  Shift Arithmetic2 : ArithShift  Commented=on  BitShiftNumber=1
  Shift Arithmetic4 : ArithShift  BitShiftNumber=8
  Sign : Signum
  Subsystem : Subsystem  Commented=on
  Sum : Sum  Inputs=-+
  Sum1 : Sum  Commented=on  Inputs=|++
  Sum2 : Sum
  Unit Delay : UnitDelay  SampleTime=-1  HasFrameUpgradeWarning=on
  atan_1 : MATLAB Function  Commented=on  TreatAsAtomicUnit=on
  ialpha{1..5} (5 alike) : InportShadow  Port=2
  ibeta{1..5} (5 alike) : InportShadow  Port=4
  obs_chart : Stateflow chart  TreatAsAtomicUnit=on
      settings: PortSchema="{\"entries\":[{\"content\":{\"sides\":[{\"content\":{\"connectorIds\":[\"In1\",\"In2\"]},\"type\":\"ConnectorPlacement.EquallySpacedRectSide\",\"uuid\":\"14a0672e-a5c3-40c4-af10-c19db619bd66\"},{\"content\":{\"connectorIds\":[\"Out1\",\"Out2\"],\"side\":\"RIGHT\"},\"type\":\"ConnectorPlacement.EquallySpacedRectSide\",\"uuid\":\"bef62292-30f4-45bd-b61f-5e325f606a28\"},{\"content\":{\"connectorIds\":[\"In3\"],\"side\":\"TOP\"},\"type\":\"ConnectorPlacement.EquallySpacedRectSide\",\"uuid\":\"f3cfe9f7-f211-4893-b433-5ed79b2485a6\"}]},\"type\":\"ConnectorPlacement.EquallySpacedConnector\",\"uuid\":\"85adbdf4-4a0a-43af-a386-f5f1a0cbbbae\"}],\"packageUris\":[\"http://schema.mathworks.com/mf0/Connector/R2020b\"],\"version\":\"1.0\"}"
  ualpha{1..4} (4 alike) : InportShadow
  ubeta{1..4} (4 alike) : InportShadow  Port=3
  提取波 : Subsystem
  浮点但是数量级是定点的NFO : Subsystem  Commented=on
  滤波器 : Subsystem
  纯浮点NFO : Subsystem  Commented=on
  Obs_Spd : Outport  OutputWhenDisabled=reset  InitialOutput=int32(0)
  Obs_Theta : Outport  Port=2  OutputWhenDisabled=reset  InitialOutput=uint16(0)
  wires:
  ualpha1/1 -> Subsystem/3(ualpha)
  ialpha1/1 -> Subsystem/6(ialpha)
  ubeta1/1 -> Subsystem/7(In7)
  ibeta1/1 -> Subsystem/8(In8)
  ualpha3/1 -> 纯浮点NFO/1(ualpha)
  ialpha3/1 -> 纯浮点NFO/2(ialpha)
  ubeta3/1 -> 纯浮点NFO/3(ubeta)
  ibeta3/1 -> 纯浮点NFO/4(ibeta)
  ualpha2/1 -> 浮点但是数量级是定点的NFO/1(ualpha)
  ialpha2/1 -> 浮点但是数量级是定点的NFO/2(ialpha)
  ubeta2/1 -> 浮点但是数量级是定点的NFO/3(ubeta)
  ibeta2/1 -> 浮点但是数量级是定点的NFO/4(ibeta)
  ualpha4/1 -> NFO/1(ualpha)
  ialpha4/1 -> NFO/2(ialpha)
  ubeta4/1 -> NFO/3(ubeta)
  ibeta4/1 -> NFO/4(ibeta)
  Udc_Ref/1 -> NFO/5(Udc_Ref)
  NFO/1(cos) -> PLL2/1(cos)
  NFO/2(sin) -> PLL2/2(sin)
  Sum1/1 -> Shift Arithmetic2/1
  ? -> Sum1/1, Delay1/1
  Delay1/1 -> Sum1/2
  ibeta5/1 -> HFI/3(ibeta)
  ialpha5/1 -> HFI/2(ialpha)
  ualpha/1 -> 提取波/1(In1)
  HF/1 -> HFI/1(HF)
  SMO/2(Ebeta) -> Scope2/2, Mux/2
  SMO/1(Ealpha) -> Scope2/1, Mux/1
  Mux1/1 -> obs_chart/2(HFI_Input)
  obs_chart/1(SMO_Output) -> Demux/1
  obs_chart/2(HFI_Output) -> Demux1/1
  [Sb] -> Scope/2  "Sb"
  [Ha] -> Scope/3  "Ha"
  Sum/1 -> PLL/1(sin)
  Sum2/1 -> Scope/1, PLL/2(cos)
  Data Store Read1/1 -> Product4/1
  Product4/1 -> Shift Arithmetic4/1
  Unit Delay/1 -> Sign/1, Abs/1
  Mux/1 -> obs_chart/1(SMO_Input)
  Demux/1 -> [Sa]
  Demux/2 -> [Sb]
  Demux1/1 -> [Hb]
  Demux1/2 -> [Ha]
  提取波/1(Out1) -> SMO/1(ualpha)
  提取波/2(Out2) -> SMO/2(ialpha)
  提取波/3(Out3) -> SMO/3(ubeta)
  提取波/4(Out4) -> SMO/4(ibeta)
  ialpha/1 -> 提取波/2(In2)
  ubeta/1 -> 提取波/3(In3)
  ibeta/1 -> 提取波/4(In4)
  PLL/1(Obs_Spd) -> Product4/2
  Shift Arithmetic4/1 -> 滤波器/1(input)
  PLL/2(Obs_Theta) -> Obs_Theta/1
  HFI/1(sin) -> Mux1/1
  HFI/2(cos) -> Mux1/2
  滤波器/1(output) -> Obs_Spd/1, Unit Delay/1
  Abs/1 -> obs_chart/3(Obs_Spd)
  Sign/1 -> SMO/5(we)
  [Sa] -> Sum/1
  [Hb] -> Sum/2
  [Sb] -> Sum2/1
  [Ha] -> Sum2/2

== system Senorless/FOC_PointModel/Park ==
  note: HFI用
  note: id = ialpha*cos(theta)+ibeta*sin(theta);
      | iq = -ialpha*sin(theta)+ibeta*cos(theta);
  ialpha : Inport
  ibeta : Inport  Port=2
  Theta_Sin : Inport  Port=3
  Theta_Cos : Inport  Port=4
  Add1 : Sum  Inputs=-+
  Add2 : Sum
  Delay1 : Delay  Commented=on  DelayLength=1
  Delay2 : Delay  DelayLength=1
  Delay3 : Delay  DelayLength=1
  Product{,1..3} (4 alike) : Product  OutDataTypeStr=int32  RndMeth=Zero
  Shift Arithmetic : ArithShift  BitShiftNumber=15  DiagnosticForOORShift=Error
  Shift Arithmetic1 : ArithShift  BitShiftNumber=15  DiagnosticForOORShift=Error
  Shift Arithmetic2 : ArithShift  Commented=on  BitShiftNumber=1
  Shift Arithmetic3 : ArithShift  BitShiftNumber=1
  Shift Arithmetic4 : ArithShift  BitShiftNumber=1
  Sum1 : Sum  Commented=on  Inputs=|++
  Sum2 : Sum  Inputs=|++
  Sum3 : Sum  Inputs=|++
  Theta_Cos1 : InportShadow  Port=4
  Theta_Sin1 : InportShadow  Port=3
  ialpha1 : InportShadow
  ibeta1 : InportShadow  Port=2
  滤波器 : Subsystem
  Id : Outport
  Iq : Outport  Port=2
  wires:
  Product1/1 -> Add2/2
  Add1/1 -> Shift Arithmetic1/1
  Add2/1 -> Shift Arithmetic/1
  Product/1 -> Add2/1
  ialpha/1 -> Product/1
  Theta_Cos/1 -> Product/2
  ibeta/1 -> Product1/1
  Theta_Sin/1 -> Product1/2
  ialpha1/1 -> Product2/1
  Theta_Sin1/1 -> Product2/2
  ibeta1/1 -> Product3/1
  Theta_Cos1/1 -> Product3/2
  Product2/1 -> Add1/1
  Product3/1 -> Add1/2
  Delay1/1 -> Sum1/2
  Sum1/1 -> Shift Arithmetic2/1
  ? -> Sum1/1, Delay1/1
  Delay2/1 -> Sum2/2
  Sum2/1 -> Shift Arithmetic3/1
  Delay3/1 -> Sum3/2
  Shift Arithmetic1/1 -> Delay3/1, Sum3/1
  Sum3/1 -> Shift Arithmetic4/1
  Shift Arithmetic/1 -> Delay2/1, Sum2/1
  Shift Arithmetic3/1 -> 滤波器/1(input)
  滤波器/1(output) -> Id/1
  Shift Arithmetic4/1 -> Iq/1

== system Senorless/FOC_PointModel/SVPWM ==
  Ualpha : Inport
  Ubeta : Inport  Port=2
  ia : Inport  Port=3
  ib : Inport  Port=4
  ic : Inport  Port=5
  AntiClark : Subsystem
  Data Store Read3 : DataStoreRead  DataStoreName=PWM_TH  IndexOptions=Index vector (dialog)  Indices=1  OutputSizes=1
  Data Store Read4 : DataStoreRead  DataStoreName=PWM_TH  IndexOptions=Index vector (dialog)  Indices=1  OutputSizes=1
  Data Type Conversion : DataTypeConversion  OutDataTypeStr=uint16  SaturateOnIntegerOverflow=off  RndMeth=Floor
  Gain1 : Gain  Gain=150e-9*36000*16384  ParamDataTypeStr=int16  OutDataTypeStr=int32  RndMeth=Zero
  Mux : Mux  Inputs=3
  Mux1 : Mux  Inputs=3
  Product : Product  OutDataTypeStr=int32  RndMeth=Zero
  Saturation : Saturate  UpperLimit=16384  LowerLimit=-16384
  Scope : Scope  NumInputPorts=2
  Shift Arithmetic : ArithShift  BitShiftNumber=1  DiagnosticForOORShift=Error
  Sign : Signum
  Sum : Sum  Inputs=++-  OutDataTypeStr=int32  RndMeth=Zero
  Sum1 : Sum  Inputs=++|  OutDataTypeStr=int16
  Sum3 : Sum  Inputs=++|  OutDataTypeStr=int32  RndMeth=Zero
  Unary Minus : UnaryMinus
  ei_t : Subsystem
  默认除以32767电压 : ArithShift  BitShiftNumber=15
  tABC : Outport
  wires:
  Ualpha/1 -> AntiClark/1(Valpha)
  Ubeta/1 -> AntiClark/2(Vbeta)
  AntiClark/1(Va) -> Mux/1
  AntiClark/2(Vb) -> Mux/2
  AntiClark/3(Vc) -> Mux/3
  Mux/1 -> ei_t/1(Vabc), Sum/2
  Data Type Conversion/1 -> tABC/1, Scope/1
  默认除以32767电压/1 -> Unary Minus/1
  Sum1/1 -> Scope/2, Data Type Conversion/1
  Data Store Read3/1 -> Shift Arithmetic/1
  Shift Arithmetic/1 -> Sum1/1
  ia/1 -> Mux1/1
  ib/1 -> Mux1/2
  ic/1 -> Mux1/3
  Mux1/1 -> Sign/1
  Sign/1 -> Gain1/1
  Product/1 -> 默认除以32767电压/1
  Data Store Read4/1 -> Product/2
  Unary Minus/1 -> Sum1/2
  Sum/1 -> Sum3/2
  Sum3/1 -> Saturation/1
  ei_t/1(ei_t) -> Sum/1
  Saturation/1 -> Product/1
